simulink model "Simulink_crazycontroller"  (Simulink 7.9)
settings: Solver=ode45  StartTime=0.0  StopTime=tspan(end)  RelTol=1e-3
PreLoadFcn:
  | warning off
  | Ts=10e-6;
InitFcn:
  | warning off
  | Ts=10e-6;
undefined symbols (not defined in the file or in its folder): sigbuilder_block
libraries: powerlib x28, powerlib_extras x2
(part 1 of 2)
PreSaveFcn:
  | warning on
settings Model: Creator=pidm  LastModifiedBy=alex  SimulationMode=accelerator
settings SolverCC: AutoInsertRateTranBlk=on
settings DataIOCC: LimitDataPoints=off  SaveFormat=StructureWithTime  SaveState=on  DSMLogging=off  InspectSignalLogs=on  ReturnWorkspaceOutputs=on  OutputOption=SpecifiedOutputTimes  OutputTimes=tspan  ReturnWorkspaceOutputsName=simout
settings RTWCC: GenCodeOnly=on  GenerateReport=on  LaunchReport=on
settings GRTTargetCC: CombineOutputUpdateFcns=off  GRTInterface=on

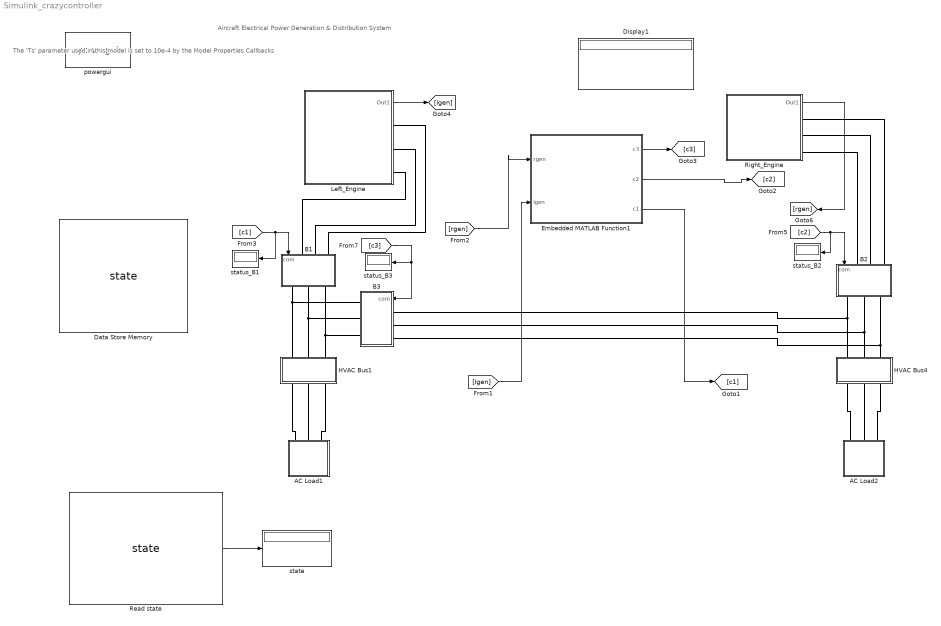
== system Simulink_crazycontroller ==
  note: The 'Ts' parameter used in this model
      | is set to 10e-4  by the Model Properties Callbacks
  note: Aircraft Electrical Power Generation & Distribution System
  AC Load1 : Subsystem
      mask Display: image(imread('power_aircraft_distribution_ACLamp.jpg','jpg'))
  AC Load2 : Subsystem
      mask Display: image(imread('power_aircraft_distribution_ACLamp.jpg','jpg'))
  B1 : Subsystem
      mask Type: Contactor
      mask Description: Simple three phase contactor without a fuse.
      mask Display:
      | plot([0.236212508752942;73.9345152396709], [85.2727156598121;85.2727156598121])
      | patch([0;170.545431319624;170.545431319624;0;0;0.472425017505884;0.472425017505884;170.073006302118;170.073006302118;0.472425017505884;0], [170.545431319624;170.545431319624;0;0;170.545431319624;170.073006302118;0.472425017505884;0.472425017505884;170.073006302118;170.073006302118;170.545431319624], [1;1;1])
      | plot([96.6109160799533;170.309218810871], [85.2727156598121;85.2727156598121])
      | patch([73.9345152396709;79.6036154497415;79.6036154497415;73.9345152396709;73.9345152396709], [119.287316920236;119.287316920236;51.2581143993884;51.2581143993884;119.287316920236], [0;0;0])
      | plot([73.9345152396709;79.6036154497415;79.6036154497415;73.9345152396709;73.9345152396709], [119.287316920236;119.287316920236;51.2581143993884;51.2581143993884;119.287316920236])
      | patch([90.9418158698827;96.6109160799533;96.6109160799533;90.9418158698827;90.9418158698827], [119.287316920236;119.287316920236;51.2581143993884;51.2581143993884;119.287316920236], [0;0;0])
      | plot([90.9418158698827;96.6109160799533;96.6109160799533;90.9418158698827;90.9418158698827], [119.287316920236;119.287316920236;51.2581143993884;51.2581143993884;119.287316920236])
      | ;
  B2 : Subsystem
      mask Type: Contactor
      mask Description: Simple three phase contactor without a fuse.
      mask Display:
      | plot([0.236212508752942;73.9345152396709], [85.2727156598121;85.2727156598121])
      | patch([0;170.545431319624;170.545431319624;0;0;0.472425017505884;0.472425017505884;170.073006302118;170.073006302118;0.472425017505884;0], [170.545431319624;170.545431319624;0;0;170.545431319624;170.073006302118;0.472425017505884;0.472425017505884;170.073006302118;170.073006302118;170.545431319624], [1;1;1])
      | plot([96.6109160799533;170.309218810871], [85.2727156598121;85.2727156598121])
      | patch([73.9345152396709;79.6036154497415;79.6036154497415;73.9345152396709;73.9345152396709], [119.287316920236;119.287316920236;51.2581143993884;51.2581143993884;119.287316920236], [0;0;0])
      | plot([73.9345152396709;79.6036154497415;79.6036154497415;73.9345152396709;73.9345152396709], [119.287316920236;119.287316920236;51.2581143993884;51.2581143993884;119.287316920236])
      | patch([90.9418158698827;96.6109160799533;96.6109160799533;90.9418158698827;90.9418158698827], [119.287316920236;119.287316920236;51.2581143993884;51.2581143993884;119.287316920236], [0;0;0])
      | plot([90.9418158698827;96.6109160799533;96.6109160799533;90.9418158698827;90.9418158698827], [119.287316920236;119.287316920236;51.2581143993884;51.2581143993884;119.287316920236])
      | ;
  B3 : Subsystem
      mask Type: Contactor
      mask Description: Simple three phase contactor without a fuse.
      mask Display:
      | plot([0.236212508752942;73.9345152396709], [85.2727156598121;85.2727156598121])
      | patch([0;170.545431319624;170.545431319624;0;0;0.472425017505884;0.472425017505884;170.073006302118;170.073006302118;0.472425017505884;0], [170.545431319624;170.545431319624;0;0;170.545431319624;170.073006302118;0.472425017505884;0.472425017505884;170.073006302118;170.073006302118;170.545431319624], [1;1;1])
      | plot([96.6109160799533;170.309218810871], [85.2727156598121;85.2727156598121])
      | patch([73.9345152396709;79.6036154497415;79.6036154497415;73.9345152396709;73.9345152396709], [119.287316920236;119.287316920236;51.2581143993884;51.2581143993884;119.287316920236], [0;0;0])
      | plot([73.9345152396709;79.6036154497415;79.6036154497415;73.9345152396709;73.9345152396709], [119.287316920236;119.287316920236;51.2581143993884;51.2581143993884;119.287316920236])
      | patch([90.9418158698827;96.6109160799533;96.6109160799533;90.9418158698827;90.9418158698827], [119.287316920236;119.287316920236;51.2581143993884;51.2581143993884;119.287316920236], [0;0;0])
      | plot([90.9418158698827;96.6109160799533;96.6109160799533;90.9418158698827;90.9418158698827], [119.287316920236;119.287316920236;51.2581143993884;51.2581143993884;119.287316920236])
      | ;
  Data Store Memory : DataStoreMemory  DataStoreName=state  ReadBeforeWriteMsg=warning  WriteAfterWriteMsg=warning  WriteAfterReadMsg=warning  OutDataTypeStr=double
  Display1 : Display
      settings: Floating=on  SampleTime=1e-2
  Embedded MATLAB Function1 : MATLAB Function  TreatAsAtomicUnit=on
  HVAC Bus1 : Subsystem
  HVAC Bus4 : Subsystem
  Left_Engine : Subsystem
      mask Display: plot(-80,-50,80,50,[0,9,18,24,29,30,29,24,18,9,0,-9,-18,-24,-29,-30,-29,-24,-18,-9,0],[30,29,24,18,9,0,-9,-18,-24,-29,-30,-29,-24,-18,-9,0,9,18,24,29,30],[-50 -30],[0 0],[50,30],[0 0],[45 35 40 40 40],[15 15 15 20 10],[1 2 3 4 5 6 7 8 9 10 11 12 13 14 15 16 17 18 19 20 21].*1.5-15,[0,9,18,24,29,30,29,24,18,9,0,-9,-18,-24,-29,-30,-29,-24,-18,-9,0]./2.4)
  Read state : DataStoreRead  DataStoreName=state
  Right_Engine : Subsystem
      mask Display: plot(-80,-50,80,50,[0,9,18,24,29,30,29,24,18,9,0,-9,-18,-24,-29,-30,-29,-24,-18,-9,0],[30,29,24,18,9,0,-9,-18,-24,-29,-30,-29,-24,-18,-9,0,9,18,24,29,30],[-50 -30],[0 0],[50,30],[0 0],[45 35 40 40 40],[15 15 15 20 10],[1 2 3 4 5 6 7 8 9 10 11 12 13 14 15 16 17 18 19 20 21].*1.5-15,[0,9,18,24,29,30,29,24,18,9,0,-9,-18,-24,-29,-30,-29,-24,-18,-9,0]./2.4)
  powergui : powerlib/powergui  SimulationMode=Discrete  SolverType=Tustin  SampleTime=Ts  frequency=60  SPID=off  DisableSnubberDevices=off  DisableRonSwitches=off  DisableVfSwitches=off  SwTol=0  Interpol=off  DisplayEquations=off  FunctionMessages=off  frequencyindice=0  Pbase=100e6  ErrMax=1e-4  Iterations=50  UnitsV=kV  UnitsW=MW  echomessages=off  HookPort=off  EnableUseOfTLC=off  x0status=blocks  RestoreLinks=warning  ResistiveCurrentMeasurement=off  Ylog=off  Xlog=on  ShowGrid=off  save=off  variable=ZData  ZoomFFT=off  StartTime=0.0  cycles=1  DisplayStyle=1  FreqAxis=off  MaxFrequency=1000  frequencyindicesteady=1  display=off  methode=off
  state : Display
  status_B1 : Display
      settings: SampleTime=1e-2
  status_B2 : Display
      settings: SampleTime=1e-2
  status_B3 : Display
      settings: SampleTime=1e-2
  wires:
  [c1] -> B1/1(com), status_B1/1
  Right_Engine/1(Out1) -> [rgen]
  [c2] -> B2/1(com), status_B2/1
  [c3] -> B3/1(com), status_B3/1
  [rgen] -> Embedded MATLAB Function1/1(rgen)
  Left_Engine/1(Out1) -> [lgen]
  [lgen] -> Embedded MATLAB Function1/2(lgen)
  Embedded MATLAB Function1/2(c2) -> [c2]
  Embedded MATLAB Function1/3(c1) -> [c1]
  Embedded MATLAB Function1/1(c3) -> [c3]
  Read state/1 -> state/1
  connections:
  Right_Engine/RConn3 -- B2/LConn1
  Left_Engine/RConn3 -- B1/LConn1
  Left_Engine/RConn2 -- B1/LConn2
  Left_Engine/RConn1 -- B1/LConn3
  B1/RConn1 -- HVAC Bus1/LConn1 -- B3/RConn1
  B1/RConn2 -- HVAC Bus1/LConn2 -- B3/RConn2
  B1/RConn3 -- HVAC Bus1/LConn3 -- B3/RConn3
  B3/LConn1 -- HVAC Bus4/LConn1 -- B2/RConn1
  B3/LConn2 -- HVAC Bus4/LConn2 -- B2/RConn2
  B3/LConn3 -- HVAC Bus4/LConn3 -- B2/RConn3
  Right_Engine/RConn2 -- B2/LConn2
  Right_Engine/RConn1 -- B2/LConn3
  HVAC Bus1/RConn1 -- AC Load1/LConn1
  HVAC Bus1/RConn2 -- AC Load1/LConn2
  HVAC Bus1/RConn3 -- AC Load1/LConn3
  HVAC Bus4/RConn1 -- AC Load2/LConn1
  HVAC Bus4/RConn2 -- AC Load2/LConn2
  HVAC Bus4/RConn3 -- AC Load2/LConn3

== system Simulink_crazycontroller/AC Load1 ==
  note: AC Load
  Iabc1 : Scope  NumInputPorts=2
      settings: TimeRange=5  YMin=-175~-8  YMax=175~8  SaveName=vdc1  SampleTime=10e-6
  Lamp 1000 Watts : powerlib/Elements/Three-Phase Series RLC Load  LConnTagsString=A|B|C  Configuration=Y (grounded)  NominalVoltage=115  NominalFrequency=400  ActivePower=1000  InductivePower=0  CapacitivePower=0  Measurements=None  LoadType=constant Z
  Three Phase  Measurement : powerlib/Measurements/Three-Phase V-I Measurement  VoltageMeasurement=phase-to-phase  SetLabelV=off  LabelV=Vabc  Vpu=off  VpuLL=off  CurrentMeasurement=yes  SetLabelI=off  LabelI=Iabc  Ipu=off  Pbase=100e6  Vbase=500e3  OutputType=Complex  PhasorSimulation=off  PSBequivalent=0
  A : PMIOPort  Port=1  Side=Left
  B : PMIOPort  Port=2  Side=Left
  C : PMIOPort  Port=3  Side=Left
  wires:
  Three Phase  Measurement/1 -> Iabc1/1  "Vac1"
  Three Phase  Measurement/2 -> Iabc1/2
  connections:
  Three Phase  Measurement/LConn2 -- B/RConn1
  Three Phase  Measurement/LConn1 -- A/RConn1
  C/RConn1 -- Three Phase  Measurement/LConn3
  Lamp 1000 Watts/LConn1 -- Three Phase  Measurement/RConn1
  Lamp 1000 Watts/LConn2 -- Three Phase  Measurement/RConn2
  Three Phase  Measurement/RConn3 -- Lamp 1000 Watts/LConn3

== system Simulink_crazycontroller/AC Load2 ==
  note: AC Load
  Iabc1 : Scope  NumInputPorts=2
      settings: TimeRange=5  YMin=-175~-20  YMax=175~17.5  SaveName=vdc3  SampleTime=10e-6
  Lamp 1000 Watts : powerlib/Elements/Three-Phase Series RLC Load  LConnTagsString=A|B|C  Configuration=Y (grounded)  NominalVoltage=115  NominalFrequency=400  ActivePower=1000  InductivePower=0  CapacitivePower=0  Measurements=None  LoadType=constant Z
  Three Phase  Measurement : powerlib/Measurements/Three-Phase V-I Measurement  VoltageMeasurement=phase-to-phase  SetLabelV=off  LabelV=Vabc  Vpu=off  VpuLL=off  CurrentMeasurement=yes  SetLabelI=off  LabelI=Iabc  Ipu=off  Pbase=100e6  Vbase=500e3  OutputType=Complex  PhasorSimulation=off  PSBequivalent=0
  A : PMIOPort  Port=1  Side=Left
  B : PMIOPort  Port=2  Side=Left
  C : PMIOPort  Port=3  Side=Left
  wires:
  Three Phase  Measurement/1 -> Iabc1/1  "Vac2"
  Three Phase  Measurement/2 -> Iabc1/2
  connections:
  Three Phase  Measurement/LConn2 -- B/RConn1
  Three Phase  Measurement/LConn1 -- A/RConn1
  C/RConn1 -- Three Phase  Measurement/LConn3
  Lamp 1000 Watts/LConn1 -- Three Phase  Measurement/RConn1
  Lamp 1000 Watts/LConn2 -- Three Phase  Measurement/RConn2
  Three Phase  Measurement/RConn3 -- Lamp 1000 Watts/LConn3

== system Simulink_crazycontroller/B1 ==
  com : Inport
  Contactor : Subsystem
  A1 : PMIOPort  Port=1  Side=Right
  B1 : PMIOPort  Port=2  Side=Right
  C1 : PMIOPort  Port=3  Side=Right
  A : PMIOPort  Port=4  Side=Left
  B : PMIOPort  Port=5  Side=Left
  C : PMIOPort  Port=6  Side=Left
  wires:
  com/1 -> Contactor/1(com)
  connections:
  Contactor/RConn1 -- A1/RConn1
  Contactor/RConn2 -- B1/RConn1
  Contactor/RConn3 -- C1/RConn1
  A/RConn1 -- Contactor/LConn1
  B/RConn1 -- Contactor/LConn2
  C/RConn1 -- Contactor/LConn3

== system Simulink_crazycontroller/B2 ==
  com : Inport
  Contactor : Subsystem
  A1 : PMIOPort  Port=1  Side=Right
  B1 : PMIOPort  Port=2  Side=Right
  C1 : PMIOPort  Port=3  Side=Right
  A : PMIOPort  Port=4  Side=Left
  B : PMIOPort  Port=5  Side=Left
  C : PMIOPort  Port=6  Side=Left
  wires:
  com/1 -> Contactor/1(com)
  connections:
  Contactor/RConn1 -- A1/RConn1
  Contactor/RConn2 -- B1/RConn1
  Contactor/RConn3 -- C1/RConn1
  A/RConn1 -- Contactor/LConn1
  B/RConn1 -- Contactor/LConn2
  C/RConn1 -- Contactor/LConn3

== system Simulink_crazycontroller/B3 ==
  com : Inport
  Contactor : Subsystem
  A1 : PMIOPort  Port=1  Side=Right
  B1 : PMIOPort  Port=2  Side=Right
  C1 : PMIOPort  Port=3  Side=Right
  A : PMIOPort  Port=4  Side=Left
  B : PMIOPort  Port=5  Side=Left
  C : PMIOPort  Port=6  Side=Left
  wires:
  com/1 -> Contactor/1(com)
  connections:
  Contactor/RConn1 -- A1/RConn1
  Contactor/RConn2 -- B1/RConn1
  Contactor/RConn3 -- C1/RConn1
  A/RConn1 -- Contactor/LConn1
  B/RConn1 -- Contactor/LConn2
  C/RConn1 -- Contactor/LConn3

== system Simulink_crazycontroller/HVAC Bus1 ==
  a : PMIOPort  Port=1  Side=Left
  b : PMIOPort  Port=2  Side=Left
  c : PMIOPort  Port=3  Side=Left
  "a " : PMIOPort  Port=4  Side=Right
  "b " : PMIOPort  Port=5  Side=Right
  "c " : PMIOPort  Port=6  Side=Right
  connections:
  b/RConn1 -- "b "/RConn1
  c/RConn1 -- "c "/RConn1
  a/RConn1 -- "a "/RConn1

== system Simulink_crazycontroller/HVAC Bus4 ==
  a : PMIOPort  Port=1  Side=Left
  b : PMIOPort  Port=2  Side=Left
  c : PMIOPort  Port=3  Side=Left
  "a " : PMIOPort  Port=4  Side=Right
  "b " : PMIOPort  Port=5  Side=Right
  "c " : PMIOPort  Port=6  Side=Right
  connections:
  b/RConn1 -- "b "/RConn1
  c/RConn1 -- "c "/RConn1
  a/RConn1 -- "a "/RConn1

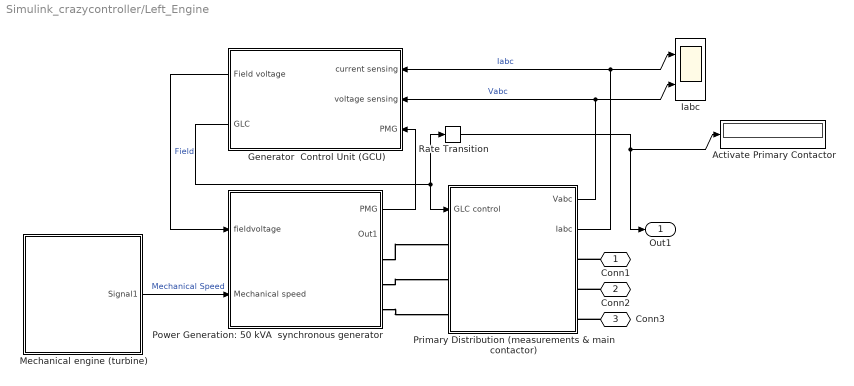
== system Simulink_crazycontroller/Left_Engine ==
  Activate Primary Contactor : Display
      settings: SampleTime=1e-2
  Generator  Control Unit (GCU) : Subsystem
      mask Display: image(imread('power_aircraft_distribution_GCU.jpg','jpg'))
  Iabc : Scope  NumInputPorts=2
      settings: TimeRange=6  YMin=-200~-300  YMax=200~300  SaveName=vac  SampleTime=10e-6
  Mechanical engine (turbine) : Subsystem  Tag=STV Subsys  LoadFcn=sigbuilder_block('load');  StartFcn=sigbuilder_block('start');  StopFcn=sigbuilder_block('stop');  ClipboardFcn=sigbuilder_block('clipboard');  mask(Sigbuilder block){}
      mask help: Sigbuilder GUI
      mask init:
      | if ~strcmp(get_param(bdroot(gcbh),'SimulationStatus'),'stopped') tuvar = sigbuilder_block('maskInit'); end
      settings: CopyFcn=sigbuilder_block('copy');  DeleteFcn=sigbuilder_block('delete');  ModelCloseFcn=sigbuilder_block('modelClose');  PreSaveFcn=sigbuilder_block('preSave');  PauseFcn=sigbuilder_block('pause')  ContinueFcn=sigbuilder_block('continue')  NameChangeFcn=sigbuilder_block('namechange');  OpenFcn=sigbuilder_block('open',[165.869 59.9528 884.303 513.595 ]);  CloseFcn=sigbuilder_block('close');
      mask Display: image(imread('power_aircraft_distribution_turbine.jpg','jpg'))
  Power Generation: 50 kVA  synchronous generator : Subsystem
      mask Display: image(imread('power_aircraft_distribution_APU_Generator.jpg','jpg'))
  Primary Distribution (measurements & main contactor) : Subsystem
  Rate Transition : RateTransition  OutPortSampleTimeOpt=Inherit  OutPortSampleTime=Ts
  Conn1 : PMIOPort  Port=1  Side=Right
  Conn2 : PMIOPort  Port=2  Side=Right
  Conn3 : PMIOPort  Port=3  Side=Right
  Out1 : Outport
  wires:
  Generator  Control Unit (GCU)/1(Field voltage) -> Power Generation: 50 kVA  synchronous generator/1(fieldvoltage)  "Field"
  Primary Distribution (measurements & main contactor)/1(Vabc) -> Generator  Control Unit (GCU)/2(voltage sensing), Iabc/2  "Vabc"
  Primary Distribution (measurements & main contactor)/2(Iabc) -> Iabc/1, Generator  Control Unit (GCU)/1(current sensing)  "Iabc"
  Generator  Control Unit (GCU)/2(GLC) -> Primary Distribution (measurements & main contactor)/1(GLC control), Rate Transition/1
  Mechanical engine (turbine)/1(Signal1) -> Power Generation: 50 kVA  synchronous generator/2(Mechanical speed)  "Mechanical Speed"
  Rate Transition/1 -> Out1/1, Activate Primary Contactor/1
  Power Generation: 50 kVA  synchronous generator/1(PMG) -> Generator  Control Unit (GCU)/3(PMG)
  connections:
  Power Generation: 50 kVA  synchronous generator/RConn1 -- Primary Distribution (measurements & main contactor)/LConn1
  Power Generation: 50 kVA  synchronous generator/RConn2 -- Primary Distribution (measurements & main contactor)/LConn2
  Power Generation: 50 kVA  synchronous generator/RConn3 -- Primary Distribution (measurements & main contactor)/LConn3
  Conn1/RConn1 -- Primary Distribution (measurements & main contactor)/RConn1
  Conn2/RConn1 -- Primary Distribution (measurements & main contactor)/RConn2
  Conn3/RConn1 -- Primary Distribution (measurements & main contactor)/RConn3

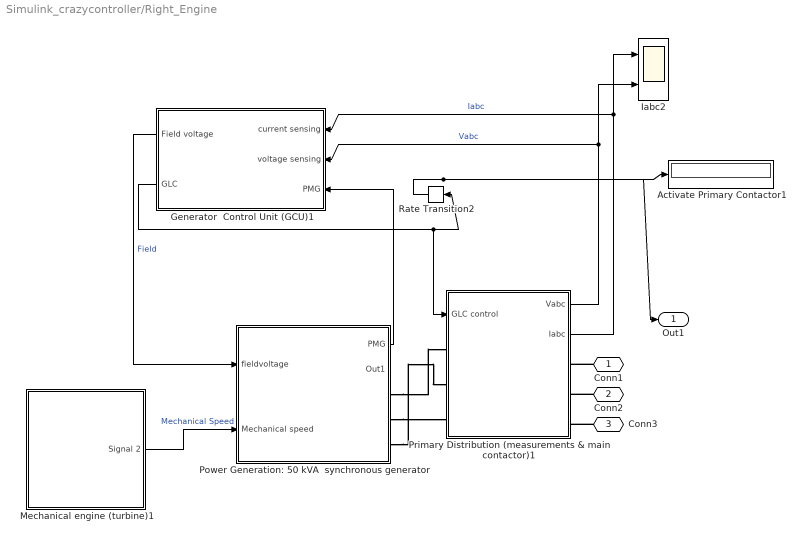
== system Simulink_crazycontroller/Right_Engine ==
  Activate Primary Contactor1 : Display
      settings: SampleTime=1e-2
  Generator  Control Unit (GCU)1 : Subsystem
      mask Display: image(imread('power_aircraft_distribution_GCU.jpg','jpg'))
  Iabc2 : Scope  NumInputPorts=2
      settings: TimeRange=6  YMin=-200~-300  YMax=200~300  SaveName=vac1  SampleTime=10e-6
  Mechanical engine (turbine)1 : Subsystem  Tag=STV Subsys  LoadFcn=sigbuilder_block('load');  StartFcn=sigbuilder_block('start');  StopFcn=sigbuilder_block('stop');  ClipboardFcn=sigbuilder_block('clipboard');  mask(Sigbuilder block){}
      mask help: Sigbuilder GUI
      mask init:
      | if ~strcmp(get_param(bdroot(gcbh),'SimulationStatus'),'stopped') tuvar = sigbuilder_block('maskInit'); end
      settings: CopyFcn=sigbuilder_block('copy');  DeleteFcn=sigbuilder_block('delete');  ModelCloseFcn=sigbuilder_block('modelClose');  PreSaveFcn=sigbuilder_block('preSave');  PauseFcn=sigbuilder_block('pause')  ContinueFcn=sigbuilder_block('continue')  NameChangeFcn=sigbuilder_block('namechange');  OpenFcn=sigbuilder_block('open',[688.457 295.767 757.403 366.711 ]);  CloseFcn=sigbuilder_block('close');
      mask Display: image(imread('power_aircraft_distribution_turbine.jpg','jpg'))
  Power Generation: 50 kVA  synchronous generator : Subsystem
      mask Display: image(imread('power_aircraft_distribution_APU_Generator.jpg','jpg'))
  Primary Distribution (measurements & main contactor)1 : Subsystem
  Rate Transition2 : RateTransition  OutPortSampleTimeOpt=Inherit  OutPortSampleTime=Ts
  Conn1 : PMIOPort  Port=1  Side=Right
  Conn2 : PMIOPort  Port=2  Side=Right
  Conn3 : PMIOPort  Port=3  Side=Right
  Out1 : Outport
  wires:
  Primary Distribution (measurements & main contactor)1/1(Vabc) -> Generator  Control Unit (GCU)1/2(voltage sensing), Iabc2/2  "Vabc"
  Primary Distribution (measurements & main contactor)1/2(Iabc) -> Iabc2/1, Generator  Control Unit (GCU)1/1(current sensing)  "Iabc"
  Generator  Control Unit (GCU)1/2(GLC) -> Primary Distribution (measurements & main contactor)1/1(GLC control), Rate Transition2/1
  Rate Transition2/1 -> Activate Primary Contactor1/1, Out1/1
  Mechanical engine (turbine)1/1(Signal 2) -> Power Generation: 50 kVA  synchronous generator/2(Mechanical speed)  "Mechanical Speed"
  Generator  Control Unit (GCU)1/1(Field voltage) -> Power Generation: 50 kVA  synchronous generator/1(fieldvoltage)  "Field"
  Power Generation: 50 kVA  synchronous generator/1(PMG) -> Generator  Control Unit (GCU)1/3(PMG)
  connections:
  Power Generation: 50 kVA  synchronous generator/RConn2 -- Primary Distribution (measurements & main contactor)1/LConn2
  Power Generation: 50 kVA  synchronous generator/RConn3 -- Primary Distribution (measurements & main contactor)1/LConn3
  Conn1/RConn1 -- Primary Distribution (measurements & main contactor)1/RConn1
  Conn2/RConn1 -- Primary Distribution (measurements & main contactor)1/RConn2
  Conn3/RConn1 -- Primary Distribution (measurements & main contactor)1/RConn3
  Power Generation: 50 kVA  synchronous generator/RConn1 -- Primary Distribution (measurements & main contactor)1/LConn1

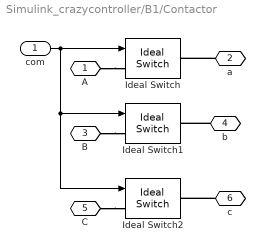
== system Simulink_crazycontroller/B1/Contactor ==
  com : Inport
  Ideal Switch : powerlib/Power Electronics/Ideal Switch  Ron=0.001  Lon=0  IC=0  Rs=1e3  Cs=inf  Measurements=off
  Ideal Switch1 : powerlib/Power Electronics/Ideal Switch  Ron=0.001  Lon=0  IC=0  Rs=1e3  Cs=inf  Measurements=off
  Ideal Switch2 : powerlib/Power Electronics/Ideal Switch  Ron=0.001  Lon=0  IC=0  Rs=1e3  Cs=inf  Measurements=off
  A : PMIOPort  Port=1  Side=Left
  a : PMIOPort  Port=2  Side=Right
  B : PMIOPort  Port=3  Side=Left
  b : PMIOPort  Port=4  Side=Right
  C : PMIOPort  Port=5  Side=Left
  c : PMIOPort  Port=6  Side=Right
  wires:
  com/1 -> Ideal Switch/1, Ideal Switch2/1, Ideal Switch1/1
  connections:
  A/RConn1 -- Ideal Switch/LConn1
  a/RConn1 -- Ideal Switch/RConn1
  B/RConn1 -- Ideal Switch1/LConn1
  b/RConn1 -- Ideal Switch1/RConn1
  C/RConn1 -- Ideal Switch2/LConn1
  c/RConn1 -- Ideal Switch2/RConn1

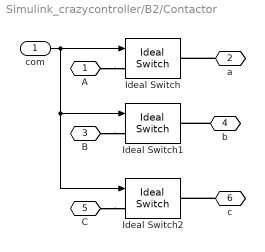
== system Simulink_crazycontroller/B2/Contactor ==
  com : Inport
  Ideal Switch : powerlib/Power Electronics/Ideal Switch  Ron=0.001  Lon=0  IC=0  Rs=1e3  Cs=inf  Measurements=off
  Ideal Switch1 : powerlib/Power Electronics/Ideal Switch  Ron=0.001  Lon=0  IC=0  Rs=1e3  Cs=inf  Measurements=off
  Ideal Switch2 : powerlib/Power Electronics/Ideal Switch  Ron=0.001  Lon=0  IC=0  Rs=1e3  Cs=inf  Measurements=off
  A : PMIOPort  Port=1  Side=Left
  a : PMIOPort  Port=2  Side=Right
  B : PMIOPort  Port=3  Side=Left
  b : PMIOPort  Port=4  Side=Right
  C : PMIOPort  Port=5  Side=Left
  c : PMIOPort  Port=6  Side=Right
  wires:
  com/1 -> Ideal Switch/1, Ideal Switch2/1, Ideal Switch1/1
  connections:
  A/RConn1 -- Ideal Switch/LConn1
  a/RConn1 -- Ideal Switch/RConn1
  B/RConn1 -- Ideal Switch1/LConn1
  b/RConn1 -- Ideal Switch1/RConn1
  C/RConn1 -- Ideal Switch2/LConn1
  c/RConn1 -- Ideal Switch2/RConn1

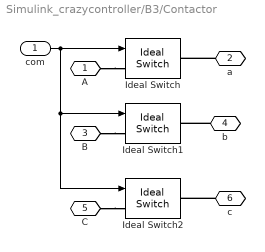
== system Simulink_crazycontroller/B3/Contactor ==
  com : Inport
  Ideal Switch : powerlib/Power Electronics/Ideal Switch  Ron=0.001  Lon=0  IC=0  Rs=1e3  Cs=inf  Measurements=off
  Ideal Switch1 : powerlib/Power Electronics/Ideal Switch  Ron=0.001  Lon=0  IC=0  Rs=1e3  Cs=inf  Measurements=off
  Ideal Switch2 : powerlib/Power Electronics/Ideal Switch  Ron=0.001  Lon=0  IC=0  Rs=1e3  Cs=inf  Measurements=off
  A : PMIOPort  Port=1  Side=Left
  a : PMIOPort  Port=2  Side=Right
  B : PMIOPort  Port=3  Side=Left
  b : PMIOPort  Port=4  Side=Right
  C : PMIOPort  Port=5  Side=Left
  c : PMIOPort  Port=6  Side=Right
  wires:
  com/1 -> Ideal Switch/1, Ideal Switch2/1, Ideal Switch1/1
  connections:
  A/RConn1 -- Ideal Switch/LConn1
  a/RConn1 -- Ideal Switch/RConn1
  B/RConn1 -- Ideal Switch1/LConn1
  b/RConn1 -- Ideal Switch1/RConn1
  C/RConn1 -- Ideal Switch2/LConn1
  c/RConn1 -- Ideal Switch2/RConn1

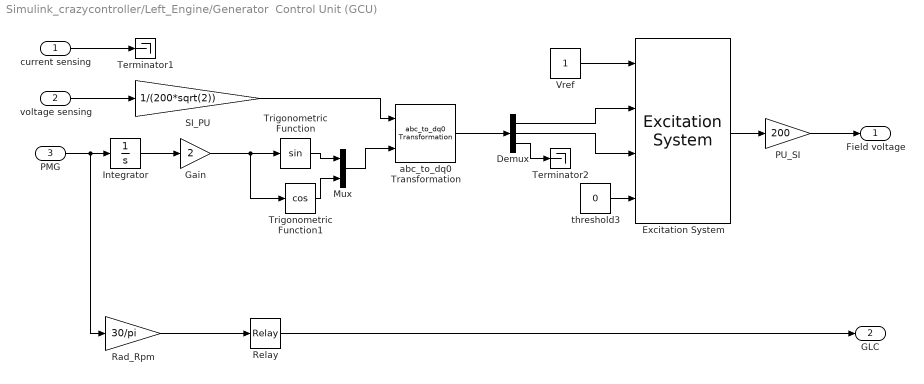
== system Simulink_crazycontroller/Left_Engine/Generator  Control Unit (GCU) ==
  current sensing : Inport
  voltage sensing : Inport  Port=2
  PMG : Inport  Port=3
  Demux : Demux  Outputs=3
  Excitation System : powerlib/Machines/Excitation System  tr=20e-3  reg=[ 300, 0.001 ]  exc=[ 1, 0 ]  tgr=[ 0, 0 ]  damp=[ 0.001, 0.1 ]  sat=[ 0, 0 ]  lim=[ -2, 2, 0 ]  v0=[1 0]
  Gain : Gain  Gain=2
  Integrator : Integrator
  Mux : Mux  Inputs=2
  PU_SI : Gain  Gain=200
  Rad_Rpm : Gain  Gain=30/pi
  Relay : Relay  OnSwitchValue=9000  OffSwitchValue=8900
  SI_PU : Gain  Gain=1/(200*sqrt(2))
  Terminator1 : Terminator
  Terminator2 : Terminator
  Trigonometric Function : Trigonometry
  Trigonometric Function1 : Trigonometry  Operator=cos
  Vref : Constant
  abc_to_dq0 Transformation : powerlib_extras/Measurements/abc_to_dq0 Transformation
  threshold3 : Constant  Value=0
  Field voltage : Outport
  GLC : Outport  Port=2
  wires:
  Relay/1 -> GLC/1
  Demux/3 -> Terminator2/1
  current sensing/1 -> Terminator1/1
  threshold3/1 -> Excitation System/4
  Vref/1 -> Excitation System/1
  Rad_Rpm/1 -> Relay/1
  PU_SI/1 -> Field voltage/1
  Excitation System/1 -> PU_SI/1
  SI_PU/1 -> abc_to_dq0 Transformation/1
  Demux/2 -> Excitation System/3
  Demux/1 -> Excitation System/2
  abc_to_dq0 Transformation/1 -> Demux/1
  Mux/1 -> abc_to_dq0 Transformation/2
  Trigonometric Function1/1 -> Mux/2
  Trigonometric Function/1 -> Mux/1
  Gain/1 -> Trigonometric Function1/1, Trigonometric Function/1
  Integrator/1 -> Gain/1
  voltage sensing/1 -> SI_PU/1
  PMG/1 -> Rad_Rpm/1, Integrator/1

== system Simulink_crazycontroller/Left_Engine/Mechanical engine (turbine) ==
  Demux : Demux  Tag=STV Demux  Outputs=1
  FromWs : FromWorkspace  Tag=STV FromWs  VariableName=tuvar  SampleTime=0  SigBuilderData=DataTag0  VnvData=DataTag1
      SigBuilderData=|
      | common.afterFinalStr = 'Extrapolate'
      | common.sampleTime = 0
      | dataSet.timeRange = [0 10]
      | dataSet.name = 'Group 1'
      | sbobj.Groups.Name = 'Group 1'
      | sbobj.Groups.Signals.Name = 'Signal1'
      | sbobj.Groups.Signals.XData = [0 1 1 1.7 1.7 2.2 2.2 2.9 2.9 3.4 3.4 4.1 4.1 4.6 4.6 5.3 5.3 5.8 5.8 6.5 6.5 7 7 7.7 7.7 8.2 8.2 8.9 8.9 9.4 9.4 10]
      | sbobj.Groups.Signals.YData = [15000 15000 15000 15000 0 0 15000 15000 0 0 15000 15000 0 0 15000 15000 0 0 15000 15000 0 0 15000 15000 0 0 15000 15000 0 0 15000 15000]
  Signal1 : Outport  Tag=STV Outport
  wires:
  FromWs/1 -> Demux/1
  Demux/1 -> Signal1/1

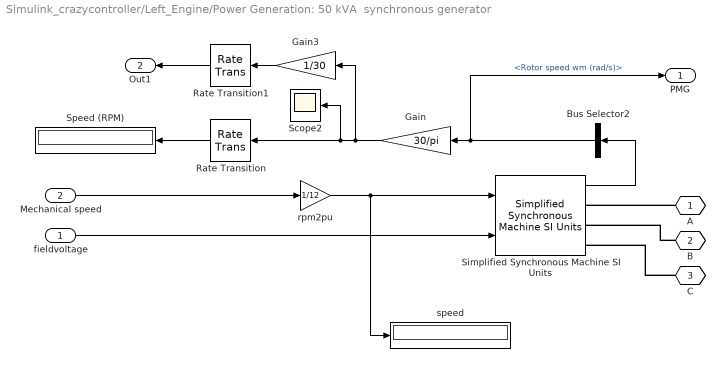
== system Simulink_crazycontroller/Left_Engine/Power Generation: 50 kVA  synchronous generator ==
  fieldvoltage : Inport
  Mechanical speed : Inport  Port=2
  Bus Selector2 : BusSelector  OutputSignals=Rotor speed wm (rad/s)
  Gain : Gain  Gain=30/pi
  Gain3 : Gain  Gain=1/30
  Rate Transition : RateTransition  OutPortSampleTimeOpt=Inherit  OutPortSampleTime=Ts
  Rate Transition1 : RateTransition  OutPortSampleTimeOpt=Inherit  OutPortSampleTime=Ts
  Scope2 : Scope
      settings: TimeRange=1  YMin=13545  YMax=13575  SaveName=ScopeData3  Decimation=100  SampleTime=1e-3
  Simplified Synchronous Machine SI Units : powerlib/Machines/Simplified Synchronous Machine SI Units  ConnectionType=3-wire Y  MechanicalLoad=Speed w  NominalParameters=[50e3 115 400]  Mechanical=[0.02 0 2]  InternalRL="[0.0204  0.08104e-3]"  InitialConditions=[-99,0 0,0,0 0,0,0]  Units=1  LoadFlowParameters=[1 0 0 0 0]  TsPowergui=0  TsBlock=-1  BusType=PV  Pref=0  Qref=0  Qmin=-inf  Qmax=+inf  PLF=0  QLF=0
  Speed (RPM) : Display
      settings: SampleTime=1e-2
  rpm2pu : Gain  Gain=1/12
  speed : Display
      settings: SampleTime=1e-2
  A : PMIOPort  Tag=PMCPort  Port=1  Side=Right
  B : PMIOPort  Tag=PMCPort  Port=2  Side=Right
  C : PMIOPort  Tag=PMCPort  Port=3  Side=Right
  PMG : Outport
  Out1 : Outport  Port=2
  wires:
  Simplified Synchronous Machine SI Units/1 -> Bus Selector2/1
  fieldvoltage/1 -> Simplified Synchronous Machine SI Units/2
  Bus Selector2/1 -> Gain/1, PMG/1  "<Rotor speed wm (rad/s)>"
  Gain/1 -> Gain3/1, Scope2/1, Rate Transition/1
  Gain3/1 -> Rate Transition1/1
  Mechanical speed/1 -> rpm2pu/1
  rpm2pu/1 -> Simplified Synchronous Machine SI Units/1, speed/1
  Rate Transition/1 -> Speed (RPM)/1
  Rate Transition1/1 -> Out1/1
  connections:
  A/RConn1 -- Simplified Synchronous Machine SI Units/RConn1
  B/RConn1 -- Simplified Synchronous Machine SI Units/RConn2
  C/RConn1 -- Simplified Synchronous Machine SI Units/RConn3

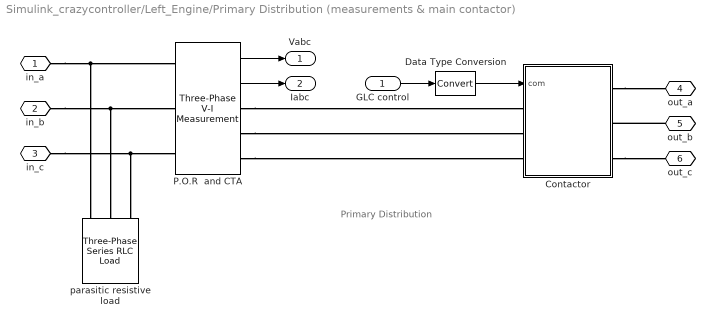
== system Simulink_crazycontroller/Left_Engine/Primary Distribution (measurements & main contactor) ==
  note: Primary Distribution
  GLC control : Inport
  Contactor : Subsystem
  Data Type Conversion : DataTypeConversion
  P.O.R  and CTA : powerlib/Measurements/Three-Phase V-I Measurement  VoltageMeasurement=phase-to-phase  SetLabelV=off  LabelV=Vabc  Vpu=off  VpuLL=off  CurrentMeasurement=yes  SetLabelI=off  LabelI=Iabc  Ipu=off  Pbase=100e6  Vbase=500e3  OutputType=Complex  PhasorSimulation=off  PSBequivalent=0
  parasitic resistive load : powerlib/Elements/Three-Phase Series RLC Load  LConnTagsString=A|B|C  Configuration=Y (grounded)  NominalVoltage=200  NominalFrequency=400  ActivePower=5000  InductivePower=0  CapacitivePower=0  Measurements=None  LoadType=constant Z
  in_a : PMIOPort  Port=1  Side=Left
  in_b : PMIOPort  Port=2  Side=Left
  in_c : PMIOPort  Port=3  Side=Left
  out_a : PMIOPort  Port=4  Side=Right
  out_b : PMIOPort  Port=5  Side=Right
  out_c : PMIOPort  Port=6  Side=Right
  Vabc : Outport
  Iabc : Outport  Port=2
  wires:
  GLC control/1 -> Data Type Conversion/1
  P.O.R  and CTA/1 -> Vabc/1
  P.O.R  and CTA/2 -> Iabc/1
  Data Type Conversion/1 -> Contactor/1(com)
  connections:
  in_a/RConn1 -- P.O.R  and CTA/LConn1 -- parasitic resistive load/LConn1
  in_b/RConn1 -- P.O.R  and CTA/LConn2 -- parasitic resistive load/LConn2
  in_c/RConn1 -- P.O.R  and CTA/LConn3 -- parasitic resistive load/LConn3
  P.O.R  and CTA/RConn1 -- Contactor/LConn1
  P.O.R  and CTA/RConn2 -- Contactor/LConn2
  P.O.R  and CTA/RConn3 -- Contactor/LConn3
  Contactor/RConn1 -- out_a/RConn1
  out_b/RConn1 -- Contactor/RConn2
  Contactor/RConn3 -- out_c/RConn1

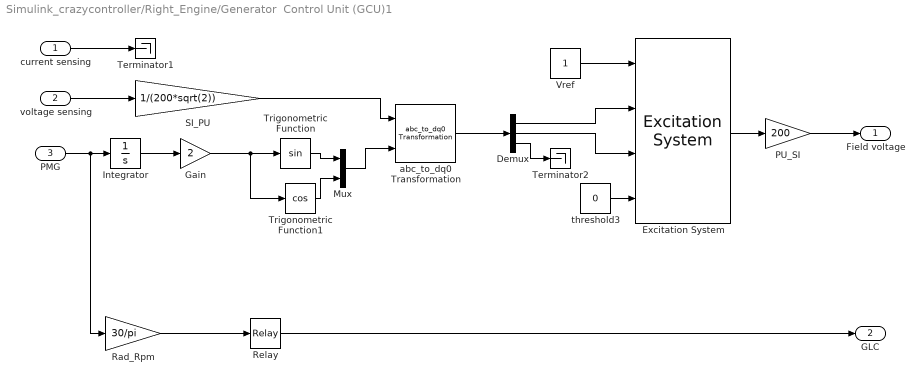
== system Simulink_crazycontroller/Right_Engine/Generator  Control Unit (GCU)1 ==
  current sensing : Inport
  voltage sensing : Inport  Port=2
  PMG : Inport  Port=3
  Demux : Demux  Outputs=3
  Excitation System : powerlib/Machines/Excitation System  tr=20e-3  reg=[ 300, 0.001 ]  exc=[ 1, 0 ]  tgr=[ 0, 0 ]  damp=[ 0.001, 0.1 ]  sat=[ 0, 0 ]  lim=[ -2, 2, 0 ]  v0=[1 0]
  Gain : Gain  Gain=2
  Integrator : Integrator
  Mux : Mux  Inputs=2
  PU_SI : Gain  Gain=200
  Rad_Rpm : Gain  Gain=30/pi
  Relay : Relay  OnSwitchValue=9000  OffSwitchValue=8900
  SI_PU : Gain  Gain=1/(200*sqrt(2))
  Terminator1 : Terminator
  Terminator2 : Terminator
  Trigonometric Function : Trigonometry
  Trigonometric Function1 : Trigonometry  Operator=cos
  Vref : Constant
  abc_to_dq0 Transformation : powerlib_extras/Measurements/abc_to_dq0 Transformation
  threshold3 : Constant  Value=0
  Field voltage : Outport
  GLC : Outport  Port=2
  wires:
  Relay/1 -> GLC/1
  Demux/3 -> Terminator2/1
  current sensing/1 -> Terminator1/1
  threshold3/1 -> Excitation System/4
  Vref/1 -> Excitation System/1
  Rad_Rpm/1 -> Relay/1
  PU_SI/1 -> Field voltage/1
  Excitation System/1 -> PU_SI/1
  SI_PU/1 -> abc_to_dq0 Transformation/1
  Demux/2 -> Excitation System/3
  Demux/1 -> Excitation System/2
  abc_to_dq0 Transformation/1 -> Demux/1
  Mux/1 -> abc_to_dq0 Transformation/2
  Trigonometric Function1/1 -> Mux/2
  Trigonometric Function/1 -> Mux/1
  Gain/1 -> Trigonometric Function1/1, Trigonometric Function/1
  Integrator/1 -> Gain/1
  voltage sensing/1 -> SI_PU/1
  PMG/1 -> Rad_Rpm/1, Integrator/1

== system Simulink_crazycontroller/Right_Engine/Mechanical engine (turbine)1 ==
  Demux : Demux  Tag=STV Demux  Outputs=1
  FromWs : FromWorkspace  Tag=STV FromWs  VariableName=tuvar  SampleTime=0  SigBuilderData=DataTag2  VnvData=DataTag3
      SigBuilderData=|
      | common.afterFinalStr = 'Extrapolate'
      | common.sampleTime = 0
      | dataSet.timeRange = [0 10]
      | dataSet.name = 'Group 1'
      | sbobj.Groups.Name = 'Group 1'
      | sbobj.Groups.Signals.Name = 'Signal 2'
      | sbobj.Groups.Signals.XData = [0 1 1 1.6 1.6 2.3 2.3 2.8 2.8 3.5 3.5 4 4 4.7 4.7 5.2 5.2 5.9 5.9 6.4 6.4 7.1 7.1 7.6 7.6 8.3 8.3 8.8 8.8 9.5 9.5 10]
      | sbobj.Groups.Signals.YData = [13800 13800 0 0 13800 13800 0 0 13800 13800 0 0 13800 13800 0 0 13800 13800 0 0 13800 13800 0 0 13800 13800 0 0 13800 13800 0 0]
  Signal 2 : Outport  Tag=STV Outport
  wires:
  FromWs/1 -> Demux/1
  Demux/1 -> Signal 2/1

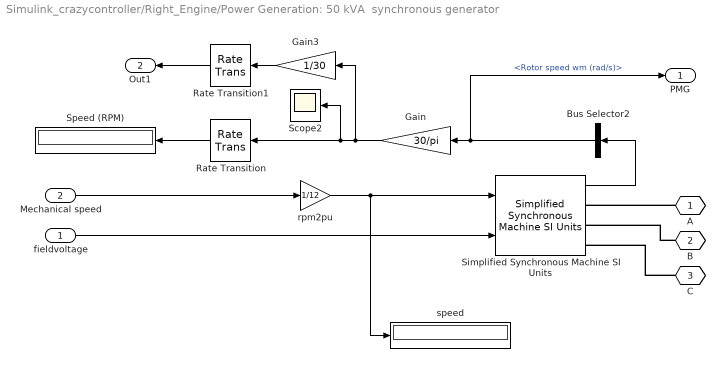
== system Simulink_crazycontroller/Right_Engine/Power Generation: 50 kVA  synchronous generator ==
  fieldvoltage : Inport
  Mechanical speed : Inport  Port=2
  Bus Selector2 : BusSelector  OutputSignals=Rotor speed wm (rad/s)
  Gain : Gain  Gain=30/pi
  Gain3 : Gain  Gain=1/30
  Rate Transition : RateTransition  OutPortSampleTimeOpt=Inherit  OutPortSampleTime=Ts
  Rate Transition1 : RateTransition  OutPortSampleTimeOpt=Inherit  OutPortSampleTime=Ts
  Scope2 : Scope
      settings: TimeRange=1  YMin=13545  YMax=13575  SaveName=ScopeData3  Decimation=100  SampleTime=1e-3
  Simplified Synchronous Machine SI Units : powerlib/Machines/Simplified Synchronous Machine SI Units  ConnectionType=3-wire Y  MechanicalLoad=Speed w  NominalParameters=[50e3 115 400]  Mechanical=[0.02 0 2]  InternalRL="[0.0204  0.08104e-3]"  InitialConditions=[-99,0 0,0,0 0,0,0]  Units=1  LoadFlowParameters=[1 0 0 0 0]  TsPowergui=0  TsBlock=-1  BusType=PV  Pref=0  Qref=0  Qmin=-inf  Qmax=+inf  PLF=0  QLF=0
  Speed (RPM) : Display
      settings: SampleTime=1e-2
  rpm2pu : Gain  Gain=1/12
  speed : Display
      settings: SampleTime=1e-2
  A : PMIOPort  Tag=PMCPort  Port=1  Side=Right
  B : PMIOPort  Tag=PMCPort  Port=2  Side=Right
  C : PMIOPort  Tag=PMCPort  Port=3  Side=Right
  PMG : Outport
  Out1 : Outport  Port=2
  wires:
  Simplified Synchronous Machine SI Units/1 -> Bus Selector2/1
  fieldvoltage/1 -> Simplified Synchronous Machine SI Units/2
  Bus Selector2/1 -> Gain/1, PMG/1  "<Rotor speed wm (rad/s)>"
  Gain/1 -> Gain3/1, Scope2/1, Rate Transition/1
  Gain3/1 -> Rate Transition1/1
  Mechanical speed/1 -> rpm2pu/1
  rpm2pu/1 -> Simplified Synchronous Machine SI Units/1, speed/1
  Rate Transition/1 -> Speed (RPM)/1
  Rate Transition1/1 -> Out1/1
  connections:
  A/RConn1 -- Simplified Synchronous Machine SI Units/RConn1
  B/RConn1 -- Simplified Synchronous Machine SI Units/RConn2
  C/RConn1 -- Simplified Synchronous Machine SI Units/RConn3

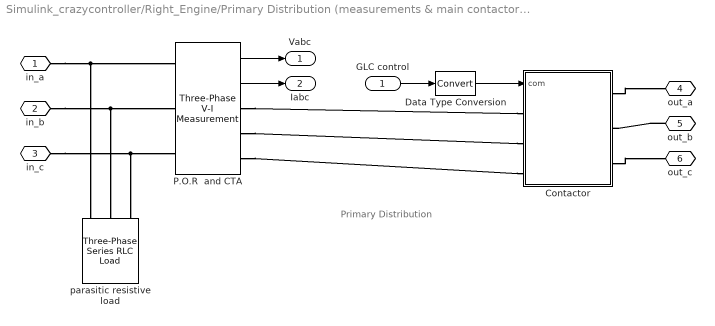
== system Simulink_crazycontroller/Right_Engine/Primary Distribution (measurements & main contactor)1 ==
  note: Primary Distribution
  GLC control : Inport
  Contactor : Subsystem
  Data Type Conversion : DataTypeConversion
  P.O.R  and CTA : powerlib/Measurements/Three-Phase V-I Measurement  VoltageMeasurement=phase-to-phase  SetLabelV=off  LabelV=Vabc  Vpu=off  VpuLL=off  CurrentMeasurement=yes  SetLabelI=off  LabelI=Iabc  Ipu=off  Pbase=100e6  Vbase=500e3  OutputType=Complex  PhasorSimulation=off  PSBequivalent=0
  parasitic resistive load : powerlib/Elements/Three-Phase Series RLC Load  LConnTagsString=A|B|C  Configuration=Y (grounded)  NominalVoltage=200  NominalFrequency=400  ActivePower=5000  InductivePower=0  CapacitivePower=0  Measurements=None  LoadType=constant Z
  in_a : PMIOPort  Port=1  Side=Left
  in_b : PMIOPort  Port=2  Side=Left
  in_c : PMIOPort  Port=3  Side=Left
  out_a : PMIOPort  Port=4  Side=Right
  out_b : PMIOPort  Port=5  Side=Right
  out_c : PMIOPort  Port=6  Side=Right
  Vabc : Outport
  Iabc : Outport  Port=2
  wires:
  GLC control/1 -> Data Type Conversion/1
  P.O.R  and CTA/1 -> Vabc/1
  P.O.R  and CTA/2 -> Iabc/1
  Data Type Conversion/1 -> Contactor/1(com)
  connections:
  in_a/RConn1 -- P.O.R  and CTA/LConn1 -- parasitic resistive load/LConn1
  in_b/RConn1 -- P.O.R  and CTA/LConn2 -- parasitic resistive load/LConn2
  in_c/RConn1 -- P.O.R  and CTA/LConn3 -- parasitic resistive load/LConn3
  P.O.R  and CTA/RConn1 -- Contactor/LConn1
  P.O.R  and CTA/RConn2 -- Contactor/LConn2
  P.O.R  and CTA/RConn3 -- Contactor/LConn3
  Contactor/RConn1 -- out_a/RConn1
  out_b/RConn1 -- Contactor/RConn2
  Contactor/RConn3 -- out_c/RConn1

== system Simulink_crazycontroller/Left_Engine/Primary Distribution (measurements & main contactor)/Contactor ==
  com : Inport
  Ideal Switch : powerlib/Power Electronics/Ideal Switch  Ron=0.001  Lon=0  IC=0  Rs=1e3  Cs=inf  Measurements=off
  Ideal Switch1 : powerlib/Power Electronics/Ideal Switch  Ron=0.001  Lon=0  IC=0  Rs=1e3  Cs=inf  Measurements=off
  Ideal Switch2 : powerlib/Power Electronics/Ideal Switch  Ron=0.001  Lon=0  IC=0  Rs=1e3  Cs=inf  Measurements=off
  A : PMIOPort  Port=1  Side=Left
  a : PMIOPort  Port=2  Side=Right
  B : PMIOPort  Port=3  Side=Left
  b : PMIOPort  Port=4  Side=Right
  C : PMIOPort  Port=5  Side=Left
  c : PMIOPort  Port=6  Side=Right
  wires:
  com/1 -> Ideal Switch1/1, Ideal Switch2/1, Ideal Switch/1
  connections:
  c/RConn1 -- Ideal Switch2/RConn1
  C/RConn1 -- Ideal Switch2/LConn1
  b/RConn1 -- Ideal Switch1/RConn1
  B/RConn1 -- Ideal Switch1/LConn1
  a/RConn1 -- Ideal Switch/RConn1
  A/RConn1 -- Ideal Switch/LConn1

== system Simulink_crazycontroller/Right_Engine/Primary Distribution (measurements & main contactor)1/Contactor ==
  com : Inport
  Ideal Switch : powerlib/Power Electronics/Ideal Switch  Ron=0.001  Lon=0  IC=0  Rs=1e3  Cs=inf  Measurements=off
  Ideal Switch1 : powerlib/Power Electronics/Ideal Switch  Ron=0.001  Lon=0  IC=0  Rs=1e3  Cs=inf  Measurements=off
  Ideal Switch2 : powerlib/Power Electronics/Ideal Switch  Ron=0.001  Lon=0  IC=0  Rs=1e3  Cs=inf  Measurements=off
  A : PMIOPort  Port=1  Side=Left
  a : PMIOPort  Port=2  Side=Right
  B : PMIOPort  Port=3  Side=Left
  b : PMIOPort  Port=4  Side=Right
  C : PMIOPort  Port=5  Side=Left
  c : PMIOPort  Port=6  Side=Right
  wires:
  com/1 -> Ideal Switch1/1, Ideal Switch2/1, Ideal Switch/1
  connections:
  c/RConn1 -- Ideal Switch2/RConn1
  C/RConn1 -- Ideal Switch2/LConn1
  b/RConn1 -- Ideal Switch1/RConn1
  B/RConn1 -- Ideal Switch1/LConn1
  a/RConn1 -- Ideal Switch/RConn1
  A/RConn1 -- Ideal Switch/LConn1
